simulink model "gm_FCS_MPC_3Phase_SPMSM_TEST1"  (R2022a)
settings: Solver=ode23t  StartTime=0.0  StopTime=0.2  RelTol=1e-3  AbsTol=1e-3  EnableMultiTasking=on
undefined symbols (not defined in the file or in its folder): f_c, Ld, Lq, np, psiPM, R, T_50MHz, u_dc
libraries: hdlmdlgenlib x26, ee_lib x22, nesl_utility x22, fl_lib x21, simulink x7
(part 5 of 5)

== system gm_FCS_MPC_3Phase_SPMSM_TEST1/Microcontroller Software/Subsystem1/MATLAB Function/square11 ==
  In1 : Inport
  In2 : Inport  Port=2
  square11 : Product  Inputs=**  OutDataTypeStr=single  SampleTime=1e-08
  Out1 : Outport
  wires:
  In1/1 -> square11/1
  In2/1 -> square11/2
  square11/1 -> Out1/1

== system gm_FCS_MPC_3Phase_SPMSM_TEST1/Microcontroller Software/Subsystem1/MATLAB Function/square12 ==
  In1 : Inport
  In2 : Inport  Port=2
  square12 : Product  Inputs=**  OutDataTypeStr=single  SampleTime=1e-08
  Out1 : Outport
  wires:
  In1/1 -> square12/1
  In2/1 -> square12/2
  square12/1 -> Out1/1

== system gm_FCS_MPC_3Phase_SPMSM_TEST1/Microcontroller Software/Subsystem1/MATLAB Function/square13 ==
  In1 : Inport
  In2 : Inport  Port=2
  square13 : Product  Inputs=**  OutDataTypeStr=single  SampleTime=1e-08
  Out1 : Outport
  wires:
  In1/1 -> square13/1
  In2/1 -> square13/2
  square13/1 -> Out1/1

== system gm_FCS_MPC_3Phase_SPMSM_TEST1/Microcontroller Software/Subsystem1/MATLAB Function/square14 ==
  In1 : Inport
  In2 : Inport  Port=2
  square14 : Product  Inputs=**  OutDataTypeStr=single  SampleTime=1e-08
  Out1 : Outport
  wires:
  In1/1 -> square14/1
  In2/1 -> square14/2
  square14/1 -> Out1/1

== system gm_FCS_MPC_3Phase_SPMSM_TEST1/Microcontroller Software/Subsystem1/MATLAB Function/square15 ==
  In1 : Inport
  In2 : Inport  Port=2
  square15 : Product  Inputs=**  OutDataTypeStr=single  SampleTime=1e-08
  Out1 : Outport
  wires:
  In1/1 -> square15/1
  In2/1 -> square15/2
  square15/1 -> Out1/1

== system gm_FCS_MPC_3Phase_SPMSM_TEST1/Microcontroller Software/Subsystem1/MATLAB Function/square2 ==
  In1 : Inport
  In2 : Inport  Port=2
  square2 : Product  Inputs=**  OutDataTypeStr=single  SampleTime=1e-08
  Out1 : Outport
  wires:
  In1/1 -> square2/1
  In2/1 -> square2/2
  square2/1 -> Out1/1

== system gm_FCS_MPC_3Phase_SPMSM_TEST1/Microcontroller Software/Subsystem1/MATLAB Function/square3 ==
  In1 : Inport
  In2 : Inport  Port=2
  square3 : Product  Inputs=**  OutDataTypeStr=single  SampleTime=1e-08
  Out1 : Outport
  wires:
  In1/1 -> square3/1
  In2/1 -> square3/2
  square3/1 -> Out1/1

== system gm_FCS_MPC_3Phase_SPMSM_TEST1/Microcontroller Software/Subsystem1/MATLAB Function/square4 ==
  In1 : Inport
  In2 : Inport  Port=2
  square4 : Product  Inputs=**  OutDataTypeStr=single  SampleTime=1e-08
  Out1 : Outport
  wires:
  In1/1 -> square4/1
  In2/1 -> square4/2
  square4/1 -> Out1/1

== system gm_FCS_MPC_3Phase_SPMSM_TEST1/Microcontroller Software/Subsystem1/MATLAB Function/square5 ==
  In1 : Inport
  In2 : Inport  Port=2
  square5 : Product  Inputs=**  OutDataTypeStr=single  SampleTime=1e-08
  Out1 : Outport
  wires:
  In1/1 -> square5/1
  In2/1 -> square5/2
  square5/1 -> Out1/1

== system gm_FCS_MPC_3Phase_SPMSM_TEST1/Microcontroller Software/Subsystem1/MATLAB Function/square6 ==
  In1 : Inport
  In2 : Inport  Port=2
  square6 : Product  Inputs=**  OutDataTypeStr=single  SampleTime=1e-08
  Out1 : Outport
  wires:
  In1/1 -> square6/1
  In2/1 -> square6/2
  square6/1 -> Out1/1

== system gm_FCS_MPC_3Phase_SPMSM_TEST1/Microcontroller Software/Subsystem1/MATLAB Function/square7 ==
  In1 : Inport
  In2 : Inport  Port=2
  square7 : Product  Inputs=**  OutDataTypeStr=single  SampleTime=1e-08
  Out1 : Outport
  wires:
  In1/1 -> square7/1
  In2/1 -> square7/2
  square7/1 -> Out1/1

== system gm_FCS_MPC_3Phase_SPMSM_TEST1/Microcontroller Software/Subsystem1/MATLAB Function/square8 ==
  In1 : Inport
  In2 : Inport  Port=2
  square8 : Product  Inputs=**  OutDataTypeStr=single  SampleTime=1e-08
  Out1 : Outport
  wires:
  In1/1 -> square8/1
  In2/1 -> square8/2
  square8/1 -> Out1/1

== system gm_FCS_MPC_3Phase_SPMSM_TEST1/Microcontroller Software/Subsystem1/MATLAB Function/square9 ==
  In1 : Inport
  In2 : Inport  Port=2
  square9 : Product  Inputs=**  OutDataTypeStr=single  SampleTime=1e-08
  Out1 : Outport
  wires:
  In1/1 -> square9/1
  In2/1 -> square9/2
  square9/1 -> Out1/1

== system gm_FCS_MPC_3Phase_SPMSM_TEST1/Microcontroller Software/Subsystem1/MATLAB Function/subtract ==
  In1 : Inport
  In2 : Inport  Port=2
  subtract : Sum  Inputs=+-  OutDataTypeStr=single  SampleTime=1e-08
  Out1 : Outport
  wires:
  In1/1 -> subtract/1
  In2/1 -> subtract/2
  subtract/1 -> Out1/1

== system gm_FCS_MPC_3Phase_SPMSM_TEST1/Microcontroller Software/Subsystem1/MATLAB Function/subtract1 ==
  In1 : Inport
  In2 : Inport  Port=2
  subtract1 : Sum  Inputs=+-  OutDataTypeStr=single  SampleTime=1e-08
  Out1 : Outport
  wires:
  In1/1 -> subtract1/1
  In2/1 -> subtract1/2
  subtract1/1 -> Out1/1

== system gm_FCS_MPC_3Phase_SPMSM_TEST1/Microcontroller Software/Subsystem1/MATLAB Function/subtract10 ==
  In1 : Inport
  In2 : Inport  Port=2
  subtract10 : Sum  Inputs=+-  OutDataTypeStr=single  SampleTime=1e-08
  Out1 : Outport
  wires:
  In1/1 -> subtract10/1
  In2/1 -> subtract10/2
  subtract10/1 -> Out1/1

== system gm_FCS_MPC_3Phase_SPMSM_TEST1/Microcontroller Software/Subsystem1/MATLAB Function/subtract11 ==
  In1 : Inport
  In2 : Inport  Port=2
  subtract11 : Sum  Inputs=+-  OutDataTypeStr=single  SampleTime=1e-08
  Out1 : Outport
  wires:
  In1/1 -> subtract11/1
  In2/1 -> subtract11/2
  subtract11/1 -> Out1/1

== system gm_FCS_MPC_3Phase_SPMSM_TEST1/Microcontroller Software/Subsystem1/MATLAB Function/subtract12 ==
  In1 : Inport
  In2 : Inport  Port=2
  subtract12 : Sum  Inputs=+-  OutDataTypeStr=single  SampleTime=1e-08
  Out1 : Outport
  wires:
  In1/1 -> subtract12/1
  In2/1 -> subtract12/2
  subtract12/1 -> Out1/1

== system gm_FCS_MPC_3Phase_SPMSM_TEST1/Microcontroller Software/Subsystem1/MATLAB Function/subtract13 ==
  In1 : Inport
  In2 : Inport  Port=2
  subtract13 : Sum  Inputs=+-  OutDataTypeStr=single  SampleTime=1e-08
  Out1 : Outport
  wires:
  In1/1 -> subtract13/1
  In2/1 -> subtract13/2
  subtract13/1 -> Out1/1

== system gm_FCS_MPC_3Phase_SPMSM_TEST1/Microcontroller Software/Subsystem1/MATLAB Function/subtract14 ==
  In1 : Inport
  In2 : Inport  Port=2
  subtract14 : Sum  Inputs=+-  OutDataTypeStr=single  SampleTime=1e-08
  Out1 : Outport
  wires:
  In1/1 -> subtract14/1
  In2/1 -> subtract14/2
  subtract14/1 -> Out1/1

== system gm_FCS_MPC_3Phase_SPMSM_TEST1/Microcontroller Software/Subsystem1/MATLAB Function/subtract15 ==
  In1 : Inport
  In2 : Inport  Port=2
  subtract15 : Sum  Inputs=+-  OutDataTypeStr=single  SampleTime=1e-08
  Out1 : Outport
  wires:
  In1/1 -> subtract15/1
  In2/1 -> subtract15/2
  subtract15/1 -> Out1/1

== system gm_FCS_MPC_3Phase_SPMSM_TEST1/Microcontroller Software/Subsystem1/MATLAB Function/subtract16 ==
  In1 : Inport
  In2 : Inport  Port=2
  subtract16 : Sum  Inputs=+-  OutDataTypeStr=single  SampleTime=1e-08
  Out1 : Outport
  wires:
  In1/1 -> subtract16/1
  In2/1 -> subtract16/2
  subtract16/1 -> Out1/1

== system gm_FCS_MPC_3Phase_SPMSM_TEST1/Microcontroller Software/Subsystem1/MATLAB Function/subtract17 ==
  In1 : Inport
  In2 : Inport  Port=2
  subtract17 : Sum  Inputs=+-  OutDataTypeStr=single  SampleTime=1e-08
  Out1 : Outport
  wires:
  In1/1 -> subtract17/1
  In2/1 -> subtract17/2
  subtract17/1 -> Out1/1

== system gm_FCS_MPC_3Phase_SPMSM_TEST1/Microcontroller Software/Subsystem1/MATLAB Function/subtract18 ==
  In1 : Inport
  In2 : Inport  Port=2
  subtract18 : Sum  Inputs=+-  OutDataTypeStr=single  SampleTime=1e-08
  Out1 : Outport
  wires:
  In1/1 -> subtract18/1
  In2/1 -> subtract18/2
  subtract18/1 -> Out1/1

== system gm_FCS_MPC_3Phase_SPMSM_TEST1/Microcontroller Software/Subsystem1/MATLAB Function/subtract19 ==
  In1 : Inport
  In2 : Inport  Port=2
  subtract19 : Sum  Inputs=+-  OutDataTypeStr=single  SampleTime=1e-08
  Out1 : Outport
  wires:
  In1/1 -> subtract19/1
  In2/1 -> subtract19/2
  subtract19/1 -> Out1/1

== system gm_FCS_MPC_3Phase_SPMSM_TEST1/Microcontroller Software/Subsystem1/MATLAB Function/subtract2 ==
  In1 : Inport
  In2 : Inport  Port=2
  subtract2 : Sum  Inputs=+-  OutDataTypeStr=single  SampleTime=1e-08
  Out1 : Outport
  wires:
  In1/1 -> subtract2/1
  In2/1 -> subtract2/2
  subtract2/1 -> Out1/1

== system gm_FCS_MPC_3Phase_SPMSM_TEST1/Microcontroller Software/Subsystem1/MATLAB Function/subtract20 ==
  In1 : Inport
  In2 : Inport  Port=2
  subtract20 : Sum  Inputs=+-  OutDataTypeStr=single  SampleTime=1e-08
  Out1 : Outport
  wires:
  In1/1 -> subtract20/1
  In2/1 -> subtract20/2
  subtract20/1 -> Out1/1

== system gm_FCS_MPC_3Phase_SPMSM_TEST1/Microcontroller Software/Subsystem1/MATLAB Function/subtract21 ==
  In1 : Inport
  In2 : Inport  Port=2
  subtract21 : Sum  Inputs=+-  OutDataTypeStr=single  SampleTime=1e-08
  Out1 : Outport
  wires:
  In1/1 -> subtract21/1
  In2/1 -> subtract21/2
  subtract21/1 -> Out1/1

== system gm_FCS_MPC_3Phase_SPMSM_TEST1/Microcontroller Software/Subsystem1/MATLAB Function/subtract22 ==
  In1 : Inport
  In2 : Inport  Port=2
  subtract22 : Sum  Inputs=+-  OutDataTypeStr=single  SampleTime=1e-08
  Out1 : Outport
  wires:
  In1/1 -> subtract22/1
  In2/1 -> subtract22/2
  subtract22/1 -> Out1/1

== system gm_FCS_MPC_3Phase_SPMSM_TEST1/Microcontroller Software/Subsystem1/MATLAB Function/subtract23 ==
  In1 : Inport
  In2 : Inport  Port=2
  subtract23 : Sum  Inputs=+-  OutDataTypeStr=single  SampleTime=1e-08
  Out1 : Outport
  wires:
  In1/1 -> subtract23/1
  In2/1 -> subtract23/2
  subtract23/1 -> Out1/1

== system gm_FCS_MPC_3Phase_SPMSM_TEST1/Microcontroller Software/Subsystem1/MATLAB Function/subtract24 ==
  In1 : Inport
  In2 : Inport  Port=2
  subtract24 : Sum  Inputs=+-  OutDataTypeStr=single  SampleTime=1e-08
  Out1 : Outport
  wires:
  In1/1 -> subtract24/1
  In2/1 -> subtract24/2
  subtract24/1 -> Out1/1

== system gm_FCS_MPC_3Phase_SPMSM_TEST1/Microcontroller Software/Subsystem1/MATLAB Function/subtract25 ==
  In1 : Inport
  In2 : Inport  Port=2
  subtract25 : Sum  Inputs=+-  OutDataTypeStr=single  SampleTime=1e-08
  Out1 : Outport
  wires:
  In1/1 -> subtract25/1
  In2/1 -> subtract25/2
  subtract25/1 -> Out1/1

== system gm_FCS_MPC_3Phase_SPMSM_TEST1/Microcontroller Software/Subsystem1/MATLAB Function/subtract26 ==
  In1 : Inport
  In2 : Inport  Port=2
  subtract26 : Sum  Inputs=+-  OutDataTypeStr=single  SampleTime=1e-08
  Out1 : Outport
  wires:
  In1/1 -> subtract26/1
  In2/1 -> subtract26/2
  subtract26/1 -> Out1/1

== system gm_FCS_MPC_3Phase_SPMSM_TEST1/Microcontroller Software/Subsystem1/MATLAB Function/subtract27 ==
  In1 : Inport
  In2 : Inport  Port=2
  subtract27 : Sum  Inputs=+-  OutDataTypeStr=single  SampleTime=1e-08
  Out1 : Outport
  wires:
  In1/1 -> subtract27/1
  In2/1 -> subtract27/2
  subtract27/1 -> Out1/1

== system gm_FCS_MPC_3Phase_SPMSM_TEST1/Microcontroller Software/Subsystem1/MATLAB Function/subtract28 ==
  In1 : Inport
  In2 : Inport  Port=2
  subtract28 : Sum  Inputs=+-  OutDataTypeStr=single  SampleTime=1e-08
  Out1 : Outport
  wires:
  In1/1 -> subtract28/1
  In2/1 -> subtract28/2
  subtract28/1 -> Out1/1

== system gm_FCS_MPC_3Phase_SPMSM_TEST1/Microcontroller Software/Subsystem1/MATLAB Function/subtract29 ==
  In1 : Inport
  In2 : Inport  Port=2
  subtract29 : Sum  Inputs=+-  OutDataTypeStr=single  SampleTime=1e-08
  Out1 : Outport
  wires:
  In1/1 -> subtract29/1
  In2/1 -> subtract29/2
  subtract29/1 -> Out1/1

== system gm_FCS_MPC_3Phase_SPMSM_TEST1/Microcontroller Software/Subsystem1/MATLAB Function/subtract3 ==
  In1 : Inport
  In2 : Inport  Port=2
  subtract3 : Sum  Inputs=+-  OutDataTypeStr=single  SampleTime=1e-08
  Out1 : Outport
  wires:
  In1/1 -> subtract3/1
  In2/1 -> subtract3/2
  subtract3/1 -> Out1/1

== system gm_FCS_MPC_3Phase_SPMSM_TEST1/Microcontroller Software/Subsystem1/MATLAB Function/subtract30 ==
  In1 : Inport
  In2 : Inport  Port=2
  subtract30 : Sum  Inputs=+-  OutDataTypeStr=single  SampleTime=1e-08
  Out1 : Outport
  wires:
  In1/1 -> subtract30/1
  In2/1 -> subtract30/2
  subtract30/1 -> Out1/1

== system gm_FCS_MPC_3Phase_SPMSM_TEST1/Microcontroller Software/Subsystem1/MATLAB Function/subtract31 ==
  In1 : Inport
  In2 : Inport  Port=2
  subtract31 : Sum  Inputs=+-  OutDataTypeStr=single  SampleTime=1e-08
  Out1 : Outport
  wires:
  In1/1 -> subtract31/1
  In2/1 -> subtract31/2
  subtract31/1 -> Out1/1

== system gm_FCS_MPC_3Phase_SPMSM_TEST1/Microcontroller Software/Subsystem1/MATLAB Function/subtract32 ==
  In1 : Inport
  In2 : Inport  Port=2
  subtract32 : Sum  Inputs=+-  OutDataTypeStr=single  SampleTime=1e-08
  Out1 : Outport
  wires:
  In1/1 -> subtract32/1
  In2/1 -> subtract32/2
  subtract32/1 -> Out1/1

== system gm_FCS_MPC_3Phase_SPMSM_TEST1/Microcontroller Software/Subsystem1/MATLAB Function/subtract33 ==
  In1 : Inport
  In2 : Inport  Port=2
  subtract33 : Sum  Inputs=+-  OutDataTypeStr=single  SampleTime=1e-08
  Out1 : Outport
  wires:
  In1/1 -> subtract33/1
  In2/1 -> subtract33/2
  subtract33/1 -> Out1/1

== system gm_FCS_MPC_3Phase_SPMSM_TEST1/Microcontroller Software/Subsystem1/MATLAB Function/subtract34 ==
  In1 : Inport
  In2 : Inport  Port=2
  subtract34 : Sum  Inputs=+-  OutDataTypeStr=single  SampleTime=1e-08
  Out1 : Outport
  wires:
  In1/1 -> subtract34/1
  In2/1 -> subtract34/2
  subtract34/1 -> Out1/1

== system gm_FCS_MPC_3Phase_SPMSM_TEST1/Microcontroller Software/Subsystem1/MATLAB Function/subtract35 ==
  In1 : Inport
  In2 : Inport  Port=2
  subtract35 : Sum  Inputs=+-  OutDataTypeStr=single  SampleTime=1e-08
  Out1 : Outport
  wires:
  In1/1 -> subtract35/1
  In2/1 -> subtract35/2
  subtract35/1 -> Out1/1

== system gm_FCS_MPC_3Phase_SPMSM_TEST1/Microcontroller Software/Subsystem1/MATLAB Function/subtract36 ==
  In1 : Inport
  In2 : Inport  Port=2
  subtract36 : Sum  Inputs=+-  OutDataTypeStr=single  SampleTime=1e-08
  Out1 : Outport
  wires:
  In1/1 -> subtract36/1
  In2/1 -> subtract36/2
  subtract36/1 -> Out1/1

== system gm_FCS_MPC_3Phase_SPMSM_TEST1/Microcontroller Software/Subsystem1/MATLAB Function/subtract37 ==
  In1 : Inport
  In2 : Inport  Port=2
  subtract37 : Sum  Inputs=+-  OutDataTypeStr=single  SampleTime=1e-08
  Out1 : Outport
  wires:
  In1/1 -> subtract37/1
  In2/1 -> subtract37/2
  subtract37/1 -> Out1/1

== system gm_FCS_MPC_3Phase_SPMSM_TEST1/Microcontroller Software/Subsystem1/MATLAB Function/subtract38 ==
  In1 : Inport
  In2 : Inport  Port=2
  subtract38 : Sum  Inputs=+-  OutDataTypeStr=single  SampleTime=1e-08
  Out1 : Outport
  wires:
  In1/1 -> subtract38/1
  In2/1 -> subtract38/2
  subtract38/1 -> Out1/1

== system gm_FCS_MPC_3Phase_SPMSM_TEST1/Microcontroller Software/Subsystem1/MATLAB Function/subtract39 ==
  In1 : Inport
  In2 : Inport  Port=2
  subtract39 : Sum  Inputs=+-  OutDataTypeStr=single  SampleTime=1e-08
  Out1 : Outport
  wires:
  In1/1 -> subtract39/1
  In2/1 -> subtract39/2
  subtract39/1 -> Out1/1

== system gm_FCS_MPC_3Phase_SPMSM_TEST1/Microcontroller Software/Subsystem1/MATLAB Function/subtract4 ==
  In1 : Inport
  In2 : Inport  Port=2
  subtract4 : Sum  Inputs=+-  OutDataTypeStr=single  SampleTime=1e-08
  Out1 : Outport
  wires:
  In1/1 -> subtract4/1
  In2/1 -> subtract4/2
  subtract4/1 -> Out1/1

== system gm_FCS_MPC_3Phase_SPMSM_TEST1/Microcontroller Software/Subsystem1/MATLAB Function/subtract40 ==
  In1 : Inport
  In2 : Inport  Port=2
  subtract40 : Sum  Inputs=+-  OutDataTypeStr=single  SampleTime=1e-08
  Out1 : Outport
  wires:
  In1/1 -> subtract40/1
  In2/1 -> subtract40/2
  subtract40/1 -> Out1/1

== system gm_FCS_MPC_3Phase_SPMSM_TEST1/Microcontroller Software/Subsystem1/MATLAB Function/subtract41 ==
  In1 : Inport
  In2 : Inport  Port=2
  subtract41 : Sum  Inputs=+-  OutDataTypeStr=single  SampleTime=1e-08
  Out1 : Outport
  wires:
  In1/1 -> subtract41/1
  In2/1 -> subtract41/2
  subtract41/1 -> Out1/1

== system gm_FCS_MPC_3Phase_SPMSM_TEST1/Microcontroller Software/Subsystem1/MATLAB Function/subtract42 ==
  In1 : Inport
  In2 : Inport  Port=2
  subtract42 : Sum  Inputs=+-  OutDataTypeStr=single  SampleTime=1e-08
  Out1 : Outport
  wires:
  In1/1 -> subtract42/1
  In2/1 -> subtract42/2
  subtract42/1 -> Out1/1

== system gm_FCS_MPC_3Phase_SPMSM_TEST1/Microcontroller Software/Subsystem1/MATLAB Function/subtract5 ==
  In1 : Inport
  In2 : Inport  Port=2
  subtract5 : Sum  Inputs=+-  OutDataTypeStr=single  SampleTime=1e-08
  Out1 : Outport
  wires:
  In1/1 -> subtract5/1
  In2/1 -> subtract5/2
  subtract5/1 -> Out1/1

== system gm_FCS_MPC_3Phase_SPMSM_TEST1/Microcontroller Software/Subsystem1/MATLAB Function/subtract6 ==
  In1 : Inport
  In2 : Inport  Port=2
  subtract6 : Sum  Inputs=+-  OutDataTypeStr=single  SampleTime=1e-08
  Out1 : Outport
  wires:
  In1/1 -> subtract6/1
  In2/1 -> subtract6/2
  subtract6/1 -> Out1/1

== system gm_FCS_MPC_3Phase_SPMSM_TEST1/Microcontroller Software/Subsystem1/MATLAB Function/subtract7 ==
  In1 : Inport
  In2 : Inport  Port=2
  subtract7 : Sum  Inputs=+-  OutDataTypeStr=single  SampleTime=1e-08
  Out1 : Outport
  wires:
  In1/1 -> subtract7/1
  In2/1 -> subtract7/2
  subtract7/1 -> Out1/1

== system gm_FCS_MPC_3Phase_SPMSM_TEST1/Microcontroller Software/Subsystem1/MATLAB Function/subtract8 ==
  In1 : Inport
  In2 : Inport  Port=2
  subtract8 : Sum  Inputs=+-  OutDataTypeStr=single  SampleTime=1e-08
  Out1 : Outport
  wires:
  In1/1 -> subtract8/1
  In2/1 -> subtract8/2
  subtract8/1 -> Out1/1

== system gm_FCS_MPC_3Phase_SPMSM_TEST1/Microcontroller Software/Subsystem1/MATLAB Function/subtract9 ==
  In1 : Inport
  In2 : Inport  Port=2
  subtract9 : Sum  Inputs=+-  OutDataTypeStr=single  SampleTime=1e-08
  Out1 : Outport
  wires:
  In1/1 -> subtract9/1
  In2/1 -> subtract9/2
  subtract9/1 -> Out1/1

== system gm_FCS_MPC_3Phase_SPMSM_TEST1/Microcontroller Software/Subsystem1/MATLAB Function1/Selector_dtc_comp_dtc_comp ==
  In1 : Inport
  Selector_dtc_comp_dtc_comp : DataTypeConversion  OutDataTypeStr=uint8  SampleTime=1e-08  SaturateOnIntegerOverflow=off  RndMeth=Floor
  Out1 : Outport
  wires:
  In1/1 -> Selector_dtc_comp_dtc_comp/1
  Selector_dtc_comp_dtc_comp/1 -> Out1/1

== system gm_FCS_MPC_3Phase_SPMSM_TEST1/Microcontroller Software/Subsystem1/MATLAB Function1/Selector_dtc_comp_dtc_comp1 ==
  In1 : Inport
  Selector_dtc_comp_dtc_comp1 : DataTypeConversion  OutDataTypeStr=uint8  SampleTime=1e-08  SaturateOnIntegerOverflow=off  RndMeth=Floor
  Out1 : Outport
  wires:
  In1/1 -> Selector_dtc_comp_dtc_comp1/1
  Selector_dtc_comp_dtc_comp1/1 -> Out1/1

== system gm_FCS_MPC_3Phase_SPMSM_TEST1/Microcontroller Software/Subsystem1/MATLAB Function1/dtc ==
  In1 : Inport
  dtc : DataTypeConversion  OutDataTypeStr=double  SampleTime=1e-08  SaturateOnIntegerOverflow=off  RndMeth=Floor
  Out1 : Outport
  wires:
  In1/1 -> dtc/1
  dtc/1 -> Out1/1

== system gm_FCS_MPC_3Phase_SPMSM_TEST1/Microcontroller Software/Subsystem1/MATLAB Function1/dtc1 ==
  In1 : Inport
  dtc1 : DataTypeConversion  OutDataTypeStr=double  SampleTime=1e-08  SaturateOnIntegerOverflow=off  RndMeth=Floor
  Out1 : Outport
  wires:
  In1/1 -> dtc1/1
  dtc1/1 -> Out1/1

== system gm_FCS_MPC_3Phase_SPMSM_TEST1/Microcontroller Software/Subsystem1/MATLAB Function1/relop ==
  In1 : Inport
  In2 : Inport  Port=2
  relop : RelationalOperator  Operator=<  OutDataTypeStr=boolean  SampleTime=1e-08  InputSameDT=off
  Out1 : Outport
  wires:
  In1/1 -> relop/1
  In2/1 -> relop/2
  relop/1 -> Out1/1

== system gm_FCS_MPC_3Phase_SPMSM_TEST1/Microcontroller Software/Subsystem1/MATLAB Function1/relop1 ==
  In1 : Inport
  In2 : Inport  Port=2
  relop1 : RelationalOperator  Operator=<  OutDataTypeStr=boolean  SampleTime=1e-08  InputSameDT=off
  Out1 : Outport
  wires:
  In1/1 -> relop1/1
  In2/1 -> relop1/2
  relop1/1 -> Out1/1

== system gm_FCS_MPC_3Phase_SPMSM_TEST1/Microcontroller Software/Subsystem1/MATLAB Function1/relop2 ==
  In1 : Inport
  In2 : Inport  Port=2
  relop2 : RelationalOperator  Operator=<  OutDataTypeStr=boolean  SampleTime=1e-08  InputSameDT=off
  Out1 : Outport
  wires:
  In1/1 -> relop2/1
  In2/1 -> relop2/2
  relop2/1 -> Out1/1

== system gm_FCS_MPC_3Phase_SPMSM_TEST1/Microcontroller Software/Subsystem1/MATLAB Function1/relop3 ==
  In1 : Inport
  In2 : Inport  Port=2
  relop3 : RelationalOperator  Operator=<  OutDataTypeStr=boolean  SampleTime=1e-08  InputSameDT=off
  Out1 : Outport
  wires:
  In1/1 -> relop3/1
  In2/1 -> relop3/2
  relop3/1 -> Out1/1

== system gm_FCS_MPC_3Phase_SPMSM_TEST1/Microcontroller Software/Subsystem1/MATLAB Function1/relop4 ==
  In1 : Inport
  In2 : Inport  Port=2
  relop4 : RelationalOperator  Operator=<  OutDataTypeStr=boolean  SampleTime=1e-08  InputSameDT=off
  Out1 : Outport
  wires:
  In1/1 -> relop4/1
  In2/1 -> relop4/2
  relop4/1 -> Out1/1

== system gm_FCS_MPC_3Phase_SPMSM_TEST1/Microcontroller Software/Subsystem1/MATLAB Function1/relop5 ==
  In1 : Inport
  In2 : Inport  Port=2
  relop5 : RelationalOperator  Operator=<  OutDataTypeStr=boolean  SampleTime=1e-08  InputSameDT=off
  Out1 : Outport
  wires:
  In1/1 -> relop5/1
  In2/1 -> relop5/2
  relop5/1 -> Out1/1

== system gm_FCS_MPC_3Phase_SPMSM_TEST1/Microcontroller Software/Subsystem1/MATLAB Function1/relop6 ==
  In1 : Inport
  In2 : Inport  Port=2
  relop6 : RelationalOperator  Operator=<  OutDataTypeStr=boolean  SampleTime=1e-08  InputSameDT=off
  Out1 : Outport
  wires:
  In1/1 -> relop6/1
  In2/1 -> relop6/2
  relop6/1 -> Out1/1

== matlab function gm_FCS_MPC_3Phase_SPMSM_TEST1/3ph_Inverter/12bit ADC ==
  data: u input; y output
function y = fcn(u)
%#codegen

y = u*4095/3.3;

== matlab function gm_FCS_MPC_3Phase_SPMSM_TEST1/3ph_Inverter/12bit ADC1 ==
  data: u input; y output
function y = fcn(u)
%#codegen

y = u*4095/3.3;

== matlab function gm_FCS_MPC_3Phase_SPMSM_TEST1/3ph_Inverter/12bit ADC2 ==
  data: u input; y output
function y = fcn(u)
%#codegen

y = u*4095/3.3;

== matlab function gm_FCS_MPC_3Phase_SPMSM_TEST1/Microcontroller Software/Subsystem/MATLAB Function ==
  data: I input; Naechste_Schaltstellung output
function Naechste_Schaltstellung = fcn(I)

% Mögliche Schaltstellungen des Umrichters
Moegliche_Schaltstellungen=[0 1 0 1 0 1;1 0 0 1 0 1;1 0 1 0 0 1;0 1 1 0 0 1;0  1 1 0 1 0;0 1 0 1 1 0;1 0 0 1 1 0;1 0 1 0 1 0];

if I==0
    I=1;
end

% Ausgegebene Schaltstellung
Naechste_Schaltstellung=(Moegliche_Schaltstellungen(I,:))';

end
